simulink model "planta"  (R2014a)
settings: Solver=ode45  StartTime=0.0  StopTime=1  RelTol=1e-3
undefined symbols (not defined in the file): g, Kd, krd, l, m
settings Model: Creator=usuario  LastModifiedBy=usuario

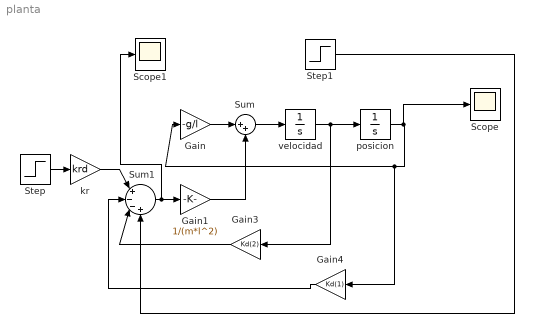
== system planta ==
  Gain : Gain  Gain=-g/l
  Gain1 : Gain  Gain=1/(m*l^2)
  Gain3 : Gain  Gain=Kd(2)
  Gain4 : Gain  Gain=Kd(1)
  Scope : Scope
  Scope1 : Scope
  Step : Step  Time=0  After=0  SampleTime=0
  Step1 : Step  Time=0  After=0  SampleTime=0
  Sum : Sum  Inputs=|++
  Sum1 : Sum  Inputs=|+--+
  kr : Gain  Gain=krd
  posicion : Integrator
  velocidad : Integrator
  wires:
  velocidad/1 -> Gain3/1, posicion/1
  posicion/1 -> Scope/1, Gain4/1, Gain/1
  Gain/1 -> Sum/1
  Sum/1 -> velocidad/1
  Gain1/1 -> Sum/2
  Step/1 -> kr/1
  Sum1/1 -> Scope1/1, Gain1/1
  kr/1 -> Sum1/1
  Gain3/1 -> Sum1/3
  Gain4/1 -> Sum1/2
  Step1/1 -> Sum1/4
